simulink model "zc_detection"  (R2019b)
settings: Solver=ode45  StartTime=0.0  StopTime=10.0  RelTol=1e-3  EnableMultiTasking=on
Description:
  | File Name:  zc_detection
  | 
  | Purpose: Zero Crossing Detection with Saturation, Switch and Abs blocks
  | 
  | Details:
  | 
  | Zero crossing detection is not limited to zero hits in signals. It also applies to sharp edges and corners in signals, as well as the saturation limits of certain block outputs.
  | 
  | If the detection of zero crossings is not significant to a simulation, you can disable it to speed up the simulation. To disable zero crossing control, set the option for Zero crossing control in the Solver pane of the Configuration Parameters dialog to Disable all.
  | 
  | You can see imperfect edges in the simulation results after the option is disabled.
settings Model: Creator=oqaqish  LastModifiedBy=khung
settings SolverCC: ZeroCrossControl=EnableAll
settings DataIOCC: LimitDataPoints=on  SaveFormat=Array  ReturnWorkspaceOutputs=off  SignalLoggingName=sigsOut
settings OptimizationCC: ExpressionDepthLimit=2147483647  InitFltsAndDblsToZero=on  LifeSpan=inf
settings DebuggingCC: SaveWithParameterizedLinksMsg=none  UnderspecifiedInitializationDetection=Classic  MergeDetectMultiDrivingBlocksExec=none  CheckExecutionContextPreStartOutputMsg=on  CheckExecutionContextRuntimeOutputMsg=on  SignalResolutionControl=TryResolveAllWithWarning  MultiTaskDSMMsg=warning  MultiTaskCondExecSysMsg=none  ParameterPrecisionLossMsg=none  FcnCallInpInsideContextMsg=warning  StateNameClashWarn=warning  SFUnexpectedBacktrackingDiag=warning  SFNoUnconditionalDefaultTransitionDiag=warning  SFExecutionAtInitializationDiag=none  ArithmeticOperatorsInVariantConditions=warning
settings HardwareCC: ProdBitPerPointer=32  ProdBitPerSizeT=32  ProdBitPerPtrDiffT=32  ProdLargestAtomicFloat=None  ProdIntDivRoundTo=Undefined  ProdEndianess=Unspecified  ProdWordSize=32  ProdHWDeviceType=32-bit Generic  TargetUnknown=on
settings ModelReferenceCC: PropagateSignalLabelsOutOfModel=off
settings SFSimCC: SimUseLocalCustomCode=off  CustomCodeUndefinedFunction=UseInterfaceOnly
settings RTWCC: RTWUseLocalCustomCode=off
settings CodeAppCC: StateflowObjectComments=on
settings GRTTargetCC: TargetFcnLib=ansi_tfl_tmw.mat  TargetLangStandard=C89/C90 (ANSI)  GeneratePreprocessorConditionals=Disable all  CombineOutputUpdateFcns=off  GRTInterface=on
settings ConfigComp: CovMetricSettings=dw  CovHtmlReporting=on  CovSaveCumulativeToWorkspaceVar=on  CovSaveSingleToWorkspaceVar=on  CovExternalEMLEnable=off

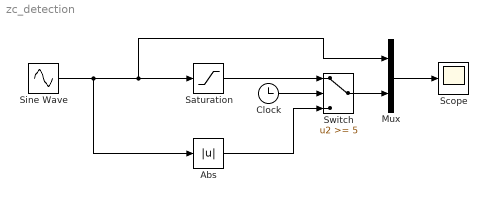
== system zc_detection ==
  Abs : Abs  SaturateOnIntegerOverflow=on
  Clock : Clock
  Mux : Mux  Inputs=2
  Saturation : Saturate  UpperLimit=2  LowerLimit=-inf
      settings: AttributesFormatString=y < %<UpperLimit>\n
  Scope : Scope
  Sine Wave : Sin  Amplitude=5  SampleTime=0
      settings: AttributesFormatString=Amplitude: %<Amplitude>
  Switch : Switch  Threshold=5  SaturateOnIntegerOverflow=on
      settings: AttributesFormatString=%<Criteria>\nThreshold = %<Threshold>
  wires:
  Sine Wave/1 -> Abs/1, Saturation/1, Mux/1
  Mux/1 -> Scope/1
  Switch/1 -> Mux/2
  Saturation/1 -> Switch/1
  Abs/1 -> Switch/3
  Clock/1 -> Switch/2
